simulink model "two_channel_no_force"  (R2019b)
settings: Solver=VariableStepAuto  StartTime=0.0  StopTime=10.0  FixedStep=0.001  RelTol=1e-3
libraries: simulink x2
settings Model: Creator=anuj  LastModifiedBy=manth

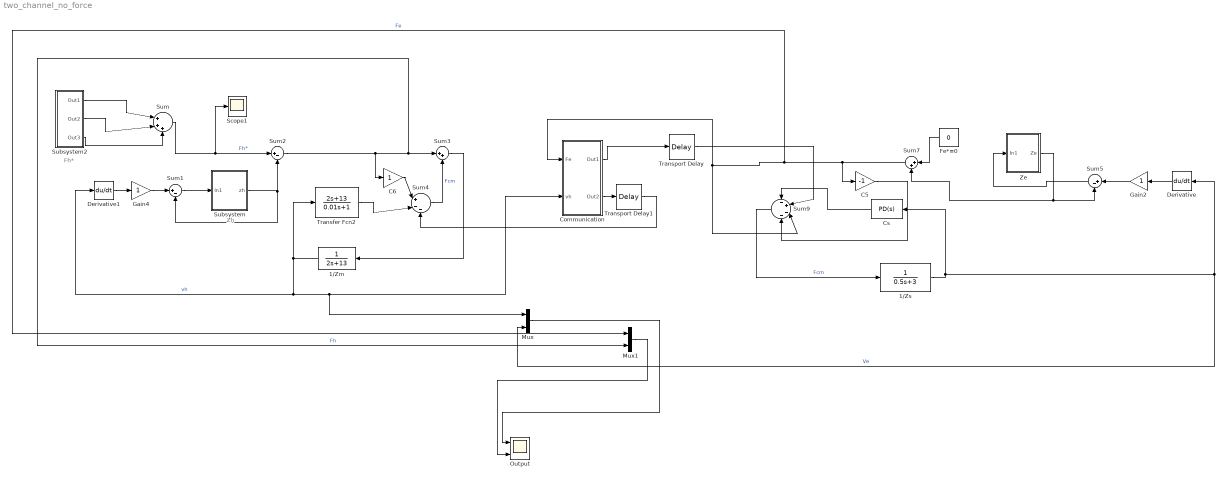
== system two_channel_no_force ==
  note: Fh*
  note: Zh
  1/Zm : TransferFcn  Denominator=[2 13]
  1/Zs : TransferFcn  Denominator=[0.5 3]
  C5 : Gain  Gain=-1
  C6 : Gain
  Communication : Subsystem
  Cs : simulink/Continuous/PID Controller  Controller=PD  Form=Parallel  TimeDomain=Continuous-time  SampleTime=-1  IntegratorMethod=Forward Euler  FilterMethod=Forward Euler  ControllerParametersSource=internal  P=1  I=1  D=1  UseFilter=on  N=1000  TunerSelectOption=Transfer Function Based (PID Tuner App)  InitialConditionSource=internal  InitialConditionForIntegrator=0  InitialConditionForFilter=0  DifferentiatorICPrevScaledInput=0  ExternalReset=none  TrackingMode=off  Kt=1  LimitOutput=off  UpperSaturationLimit=inf  LowerSaturationLimit=-inf  LinearizeAsGain=on  AntiWindupMode=none  Kb=1  POutMin=[]  POutMax=[]  IOutMin=[]  IOutMax=[]  DOutMin=[]  DOutMax=[]  NOutMin=[]  NOutMax=[]  SumOutMin=[]  SumOutMax=[]  SaturationOutMin=[]  SaturationOutMax=[]  PParamMin=[]  PParamMax=[]  IParamMin=[]  IParamMax=[]  DParamMin=[]  DParamMax=[]  NParamMin=[]  NParamMax=[]  KbParamMin=[]  KbParamMax=[]  KtParamMin=[]  KtParamMax=[]  KbOutMin=[]  KbOutMax=[]  KtOutMin=[]  KtOutMax=[]  IntegratorOutMin=[]  IntegratorOutMax=[]  FilterOutMin=[]  FilterOutMax=[]  SumI1OutMin=[]  SumI1OutMax=[]  SumI2OutMin=[]  SumI2OutMax=[]  SumI3OutMin=[]  SumI3OutMax=[]  SumI4OutMin=[]  SumI4OutMax=[]  SumDOutMin=[]  SumDOutMax=[]  DifferentiatorOutMin=[]  DifferentiatorOutMax=[]  FilterDiffOutCoefMin=[]  FilterDiffOutCoefMax=[]  ReciprocalOutMin=[]  ReciprocalOutMax=[]  SumDenOutMin=[]  SumDenOutMax=[]  SumNumOutMin=[]  SumNumOutMax=[]  DivideOutMin=[]  DivideOutMax=[]  IntegratorContinuousStateAttributes=''  IntegratorStateMustResolveToSignalObject=off  IntegratorRTWStateStorageClass=Auto  FilterContinuousStateAttributes=''  FilterStateMustResolveToSignalObject=off  FilterRTWStateStorageClass=Auto  ParallelPVariant=InternalParameters  IdealPVariant=Disabled  IVariant=Disabled  DVariant=InternalParameters  IntegratorVariant=Disabled  SatVariant=Disabled  AWVariant=Disabled  PCopyVariant=Disabled  TRVariant=Disabled  FdbkBlocksVariant=Forward  IdealPFdbkVariant=Disabled  SatFdbkVariant=Disabled  DerivativeFilterVariant=ContFilter  NVariant=InternalParameters  NCopyVariant=Disabled  FilterICVariant=InternalICsFilter  IntegratorICVariant=Disabled  ExternalResetVariant=Disabled  TRSumVariant=Passthrough  SumFdbkVariant=Disabled  SumVariant=Sum_PD
  Derivative : Derivative
  Derivative1 : Derivative
  Fe*=0 : Constant  Value=0
  Gain2 : Gain
  Gain4 : Gain
  Mux : Mux  Inputs=2
  Mux1 : Mux  Inputs=2
  Output : Scope  NumInputPorts=2
  Scope1 : Scope
  Subsystem : Subsystem
  Subsystem2 : Subsystem
  Sum : Sum  Inputs=|+++
  Sum1 : Sum  Inputs=|+-
  Sum2 : Sum  Inputs=|+-
  Sum3 : Sum  Inputs=|++
  Sum4 : Sum  Inputs=|+--
  Sum5 : Sum  Inputs=|+-
  Sum7 : Sum  Inputs=|++
  Sum9 : Sum  Inputs=-+--
  Transfer Fcn2 : TransferFcn  Numerator=[2 13]  Denominator=[0.01 1]
  Transport Delay : TransportDelay  DelayTime=0.1
  Transport Delay1 : TransportDelay  DelayTime=0.1
  Ze : Subsystem
  wires:
  Transfer Fcn2/1 -> Sum4/2
  Sum2/1 -> C6/1, Sum3/1, Mux1/2  "Fh"
  Sum7/1 -> C5/1, Mux1/1, Sum9/3, Communication/1(Fe)  "Fe"
  Sum/1 -> Scope1/1, Sum2/1  "Fh*"
  1/Zm/1 -> Transfer Fcn2/1, Derivative1/1, Communication/2(vh), Mux/1  "vh"
  Cs/1 -> Sum9/1
  Fe*=0/1 -> Sum7/1
  Sum4/1 -> Sum3/2  "Fcm"
  1/Zs/1 -> Derivative/1, Mux/2, Cs/1  "Ve"
  Sum9/1 -> 1/Zs/1  "Fcm"
  Sum3/1 -> 1/Zm/1
  Mux/1 -> Output/1
  Mux1/1 -> Output/2
  Derivative/1 -> Gain2/1
  Gain2/1 -> Sum5/1
  Gain4/1 -> Sum1/1
  Derivative1/1 -> Gain4/1
  Subsystem/1(zh) -> Sum2/2, Sum1/2
  Sum1/1 -> Subsystem/1(In1)
  Ze/1(Ze) -> Sum7/2, Sum5/2
  Sum5/1 -> Ze/1(In1)
  Subsystem2/1(Out1) -> Sum/1
  Subsystem2/2(Out2) -> Sum/2
  Subsystem2/3(Out3) -> Sum/3
  Communication/2(Out2) -> Transport Delay1/1
  Transport Delay1/1 -> Sum4/3
  Communication/1(Out1) -> Transport Delay/1
  Transport Delay/1 -> Sum9/2
  C6/1 -> Sum4/1
  C5/1 -> Sum9/4

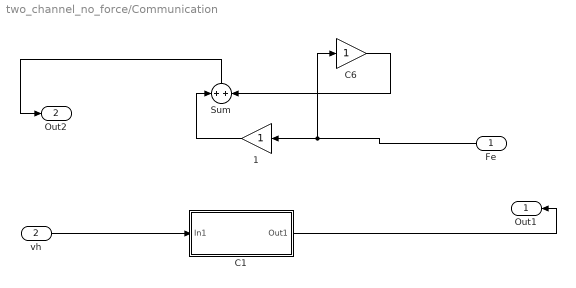
== system two_channel_no_force/Communication ==
  Fe : Inport
  vh : Inport  Port=2
  1 : Gain
  C1 : Subsystem
  C6 : Gain
  Sum : Sum
  Out1 : Outport
  Out2 : Outport  Port=2
  wires:
  Fe/1 -> C6/1, 1/1
  vh/1 -> C1/1(In1)
  C1/1(Out1) -> Out1/1
  1/1 -> Sum/1
  C6/1 -> Sum/2
  Sum/1 -> Out2/1

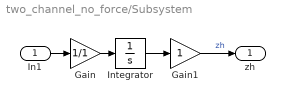
== system two_channel_no_force/Subsystem ==
  In1 : Inport
  Gain : Gain  Gain=1/1
  Gain1 : Gain
  Integrator : Integrator
  zh : Outport
  wires:
  Gain1/1 -> zh/1  "zh"
  Integrator/1 -> Gain1/1
  Gain/1 -> Integrator/1
  In1/1 -> Gain/1

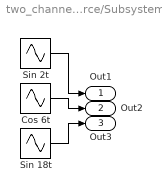
== system two_channel_no_force/Subsystem2 ==
  "Cos 6t " : Sin  Frequency=6  Phase=pi/2  SampleTime=0
  Sin 18t : Sin  Frequency=18  SampleTime=0
  Sin 2t : Sin  Frequency=2  SampleTime=0
  Out1 : Outport
  Out2 : Outport  Port=2
  Out3 : Outport  Port=3
  wires:
  Sin 2t/1 -> Out1/1
  Sin 18t/1 -> Out3/1
  "Cos 6t "/1 -> Out2/1

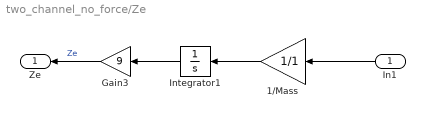
== system two_channel_no_force/Ze ==
  In1 : Inport
  1/Mass : Gain  Gain=1/1
  Gain3 : Gain  Gain=9
  Integrator1 : Integrator
  Ze : Outport
  wires:
  1/Mass/1 -> Integrator1/1
  In1/1 -> 1/Mass/1
  Integrator1/1 -> Gain3/1
  Gain3/1 -> Ze/1  "Ze"

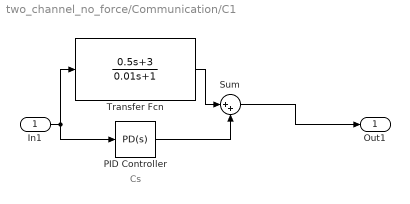
== system two_channel_no_force/Communication/C1 ==
  note: Cs
  In1 : Inport
  PID Controller : simulink/Continuous/PID Controller  Controller=PD  Form=Parallel  TimeDomain=Continuous-time  SampleTime=-1  IntegratorMethod=Forward Euler  FilterMethod=Forward Euler  ControllerParametersSource=internal  P=1  I=1  D=1  UseFilter=on  N=1000  TunerSelectOption=Transfer Function Based (PID Tuner App)  InitialConditionSource=internal  InitialConditionForIntegrator=0  InitialConditionForFilter=0  DifferentiatorICPrevScaledInput=0  ExternalReset=none  TrackingMode=off  Kt=1  LimitOutput=off  UpperSaturationLimit=inf  LowerSaturationLimit=-inf  LinearizeAsGain=on  AntiWindupMode=none  Kb=1  POutMin=[]  POutMax=[]  IOutMin=[]  IOutMax=[]  DOutMin=[]  DOutMax=[]  NOutMin=[]  NOutMax=[]  SumOutMin=[]  SumOutMax=[]  SaturationOutMin=[]  SaturationOutMax=[]  PParamMin=[]  PParamMax=[]  IParamMin=[]  IParamMax=[]  DParamMin=[]  DParamMax=[]  NParamMin=[]  NParamMax=[]  KbParamMin=[]  KbParamMax=[]  KtParamMin=[]  KtParamMax=[]  KbOutMin=[]  KbOutMax=[]  KtOutMin=[]  KtOutMax=[]  IntegratorOutMin=[]  IntegratorOutMax=[]  FilterOutMin=[]  FilterOutMax=[]  SumI1OutMin=[]  SumI1OutMax=[]  SumI2OutMin=[]  SumI2OutMax=[]  SumI3OutMin=[]  SumI3OutMax=[]  SumI4OutMin=[]  SumI4OutMax=[]  SumDOutMin=[]  SumDOutMax=[]  DifferentiatorOutMin=[]  DifferentiatorOutMax=[]  FilterDiffOutCoefMin=[]  FilterDiffOutCoefMax=[]  ReciprocalOutMin=[]  ReciprocalOutMax=[]  SumDenOutMin=[]  SumDenOutMax=[]  SumNumOutMin=[]  SumNumOutMax=[]  DivideOutMin=[]  DivideOutMax=[]  IntegratorContinuousStateAttributes=''  IntegratorStateMustResolveToSignalObject=off  IntegratorRTWStateStorageClass=Auto  FilterContinuousStateAttributes=''  FilterStateMustResolveToSignalObject=off  FilterRTWStateStorageClass=Auto  ParallelPVariant=InternalParameters  IdealPVariant=Disabled  IVariant=Disabled  DVariant=InternalParameters  IntegratorVariant=Disabled  SatVariant=Disabled  AWVariant=Disabled  PCopyVariant=Disabled  TRVariant=Disabled  FdbkBlocksVariant=Forward  IdealPFdbkVariant=Disabled  SatFdbkVariant=Disabled  DerivativeFilterVariant=ContFilter  NVariant=InternalParameters  NCopyVariant=Disabled  FilterICVariant=InternalICsFilter  IntegratorICVariant=Disabled  ExternalResetVariant=Disabled  TRSumVariant=Passthrough  SumFdbkVariant=Disabled  SumVariant=Sum_PD
  Sum : Sum  Inputs=|++
  Transfer Fcn : TransferFcn  Numerator=[0.5 3]  Denominator=[0.01 1]
  Out1 : Outport
  wires:
  In1/1 -> PID Controller/1, Transfer Fcn/1
  PID Controller/1 -> Sum/2
  Transfer Fcn/1 -> Sum/1
  Sum/1 -> Out1/1
